simulink model "sistema_caotico"  (R2025b)
settings: Solver=ode4  StartTime=0.0  StopTime=5600  FixedStep=0.01  RelTol=1e-3
settings Model: Creator=Magallón  LastModifiedBy=aleja
settings SolverCC: AlgebraicLoopSolver=TrustRegion
settings OptimizationCC: ReuseModelBlockBuffer=off
settings DebuggingCC: UnconnectedInputMsg=warning  UnconnectedOutputMsg=warning  UnconnectedLineMsg=warning
settings ModelReferenceCC: EnableRefExpFcnMdlSchedulingChecks=on
settings SFSimCC: CustomCodeUndefinedFunction=UseInterfaceOnly
settings RTWCC: GPUComputeCapability=3.5

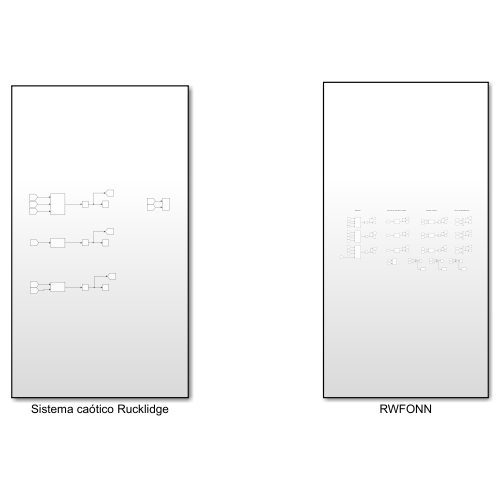
[thumbnail: Simulink's stored preview of the top-level diagram]
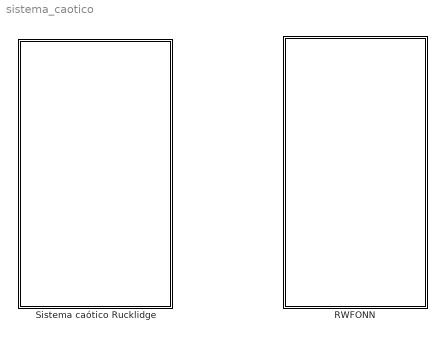
== system sistema_caotico ==
  RWFONN : Subsystem
  Sistema caótico Rucklidge : Subsystem

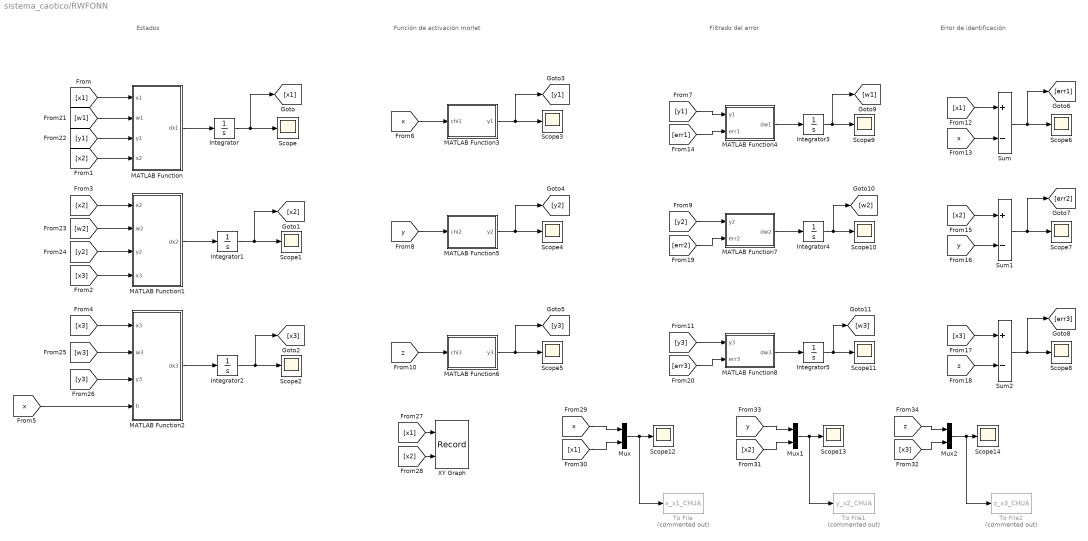
== system sistema_caotico/RWFONN ==
  note: Estados
  note: Función de activación morlet
  note: Filtrado del error
  note: Error de identificación
  Integrator : Integrator  InitialCondition=0.15
  Integrator1 : Integrator  InitialCondition=0.18
  Integrator2 : Integrator  InitialCondition=0.2
  Integrator3 : Integrator
  Integrator4 : Integrator
  Integrator5 : Integrator
  MATLAB Function : MATLAB Function  TreatAsAtomicUnit=on
  MATLAB Function1 : MATLAB Function  TreatAsAtomicUnit=on
  MATLAB Function2 : MATLAB Function  TreatAsAtomicUnit=on
  MATLAB Function3 : MATLAB Function  TreatAsAtomicUnit=on
  MATLAB Function4 : MATLAB Function  TreatAsAtomicUnit=on
  MATLAB Function5 : MATLAB Function  TreatAsAtomicUnit=on
  MATLAB Function6 : MATLAB Function  TreatAsAtomicUnit=on
  MATLAB Function7 : MATLAB Function  TreatAsAtomicUnit=on
  MATLAB Function8 : MATLAB Function  TreatAsAtomicUnit=on
  Mux : Mux  Inputs=2
  Mux1 : Mux  Inputs=2
  Mux2 : Mux  Inputs=2
  Scope{,1..14} (15 alike) : Scope
      Scope settings: ActiveDisplayYMinimum=-3.64404  ActiveDisplayYMaximum=3.74396  DataLoggingVariableName=ScopeData2
      Scope1 settings: ActiveDisplayYMinimum=-0.62184  ActiveDisplayYMaximum=0.61899  DataLoggingVariableName=ScopeData3
      Scope10 settings: DataLoggingVariableName=ScopeData8
      Scope11 settings: DataLoggingVariableName=ScopeData9
      Scope12 settings: ActiveDisplayYMinimum=-12.72999233304083  ActiveDisplayYMaximum=12.691522590822398  DataLoggingVariableName=ScopeData10
      Scope13 settings: ActiveDisplayYMinimum=-1.93605  ActiveDisplayYMaximum=1.07127  DataLoggingVariableName=ScopeData11
      Scope14 settings: ActiveDisplayYMinimum=-0.11038  ActiveDisplayYMaximum=0.33307  DataLoggingVariableName=ScopeData12
      Scope2 settings: ActiveDisplayYMinimum=-9.41356  ActiveDisplayYMaximum=31.13321  DataLoggingVariableName=ScopeData4
      Scope3 settings: ActiveDisplayYMinimum=0.95913  ActiveDisplayYMaximum=1.00454
      Scope4 settings: DataLoggingVariableName=ScopeData2
      Scope5 settings: DataLoggingVariableName=ScopeData3
      Scope6 settings: ActiveDisplayYMinimum=-0.066577278149702268  ActiveDisplayYMaximum=0.0653822169395355  DataLoggingVariableName=ScopeData4
      Scope7 settings: ActiveDisplayYMinimum=-0.00783  ActiveDisplayYMaximum=0.00738  DataLoggingVariableName=ScopeData5
      Scope8 settings: ActiveDisplayYMinimum=-1.2415250279876853  ActiveDisplayYMaximum=1.9808572797287463  DataLoggingVariableName=ScopeData6
      Scope9 settings: ActiveDisplayYMinimum=-1.38218  ActiveDisplayYMaximum=2.36611  DataLoggingVariableName=ScopeData7
  Sum : Sum  Inputs=+-
  Sum1 : Sum  Inputs=+-
  Sum2 : Sum  Inputs=+-
  To File : ToFile  Commented=on  Filename=x_x1_CHUA  MatrixName=x_x1_CHUA
  To File1 : ToFile  Commented=on  Filename=y_x2_CHUA  MatrixName=y_x2_CHUA
  To File2 : ToFile  Commented=on  Filename=z_x3_CHUA  MatrixName=z_x3_CHUA
  XY Graph : Record  NumPorts=2.0  FileSettingsInternal="{\"entries\":[{\"content\":{\"excelSettings\":{\"content\":{},\"type\":\"Streamout.ExcelSettings\"},\"parquetSettings\":{\"content\":{},\"type\":\"Streamout.ParquetSettings\"}},\"type\":\"Streamout.FileSettingStorage\",\"uuid\":\"\"}],\"packageUris\":[\"http:\\/\\/schema.mathworks.com\\/mf0\\/streamout_blocks\\/R2020a\"],\"version\":\"1.0\"}"  FrameSettings=[0, 0]  Layout=[1 1]  SignalsInternal="{\"entries\":[{\"content\":{\"signals\":[{\"content\":{\"blockPath\":[],\"dimensions\":[1],\"domain\":\"\",\"lineColor\":\"#a2142f\",\"plots\":[ 1 ],\"port\":1,\"signalID\":1,\"signalName\":\"From27\"},\"type\":\"RecordBlkView.Signal\",\"uuid\":\"\"},{\"content\":{\"blockPath\":[],\"dimensions\":[1],\"domain\":\"\",\"lineColor\":\"#139fff\",\"plots\":[ 1 ],\"port\":2,\"signalID\":2,\"signalName\":\"From28\"},\"type\":\"RecordBlkView.Signal\",\"uuid\":\"\"}]},\"type\":\"RecordBlkView.InputSignals\",\"uuid\":\"\"}],\"packageUris\":[\"http:\\/\\/schema.mathworks.com\\/mf0\\/streamout_blocks\\/R2020a\"],\"version\":\"1.0\"}"  VisualizationBindings="{\"xyplotplugin\":{\"info\":[{\"series\":[{\"bindingParametersList\":[{\"parameter\":\"X-Axis\",\"signalID\":1,\"signalName\":\"From27\"},{\"parameter\":\"Y-Axis\",\"signalID\":2,\"signalName\":\"From28\"}],\"seriesID\":0}],\"subplotID\":1}]}}"  CompatibilityTag=XY
  wires:
  MATLAB Function/1(dx1) -> Integrator/1
  MATLAB Function1/1(dx2) -> Integrator1/1
  MATLAB Function2/1(dx3) -> Integrator2/1
  Integrator/1 -> [x1], Scope/1
  Integrator1/1 -> [x2], Scope1/1
  Integrator2/1 -> [x3], Scope2/1
  [x1] -> MATLAB Function/1(x1)
  [x2] -> MATLAB Function/4(x2)
  [x3] -> MATLAB Function1/4(x3)
  [x2] -> MATLAB Function1/1(x2)
  [x3] -> MATLAB Function2/1(x3)
  MATLAB Function3/1(y1) -> [y1], Scope3/1
  [y1] -> MATLAB Function4/1(y1)
  MATLAB Function5/1(y2) -> Scope4/1, [y2]
  MATLAB Function6/1(y3) -> [y3], Scope5/1
  [y2] -> MATLAB Function7/1(y2)
  [y3] -> MATLAB Function8/1(y3)
  [x1] -> Sum/1
  Sum/1 -> [err1], Scope6/1
  [err1] -> MATLAB Function4/2(err1)
  Sum1/1 -> Scope7/1, [err2]
  [x2] -> Sum1/1
  [x3] -> Sum2/1
  Sum2/1 -> [err3], Scope8/1
  [err2] -> MATLAB Function7/2(err2)
  [err3] -> MATLAB Function8/2(err3)
  MATLAB Function4/1(dw1) -> Integrator3/1
  MATLAB Function7/1(dw2) -> Integrator4/1
  MATLAB Function8/1(dw3) -> Integrator5/1
  Integrator3/1 -> [w1], Scope9/1
  Integrator4/1 -> [w2], Scope10/1
  Integrator5/1 -> [w3], Scope11/1
  [w1] -> MATLAB Function/2(w1)
  [y1] -> MATLAB Function/3(y1)
  [w2] -> MATLAB Function1/2(w2)
  [y2] -> MATLAB Function1/3(y2)
  [w3] -> MATLAB Function2/2(w3)
  [y3] -> MATLAB Function2/3(y3)
  [x] -> Mux/1
  [x1] -> Mux/2
  Mux/1 -> To File/1, Scope12/1
  Mux1/1 -> To File1/1, Scope13/1
  [x2] -> Mux1/2
  [y] -> Mux1/1
  [z] -> Mux2/1
  [x3] -> Mux2/2
  Mux2/1 -> To File2/1, Scope14/1
  [x] -> Sum/2
  [y] -> Sum1/2
  [z] -> Sum2/2
  [x] -> MATLAB Function3/1(chi1)
  [y] -> MATLAB Function5/1(chi2)
  [z] -> MATLAB Function6/1(chi3)
  [x] -> MATLAB Function2/4(b)
  [x1] -> XY Graph/1
  [x2] -> XY Graph/2

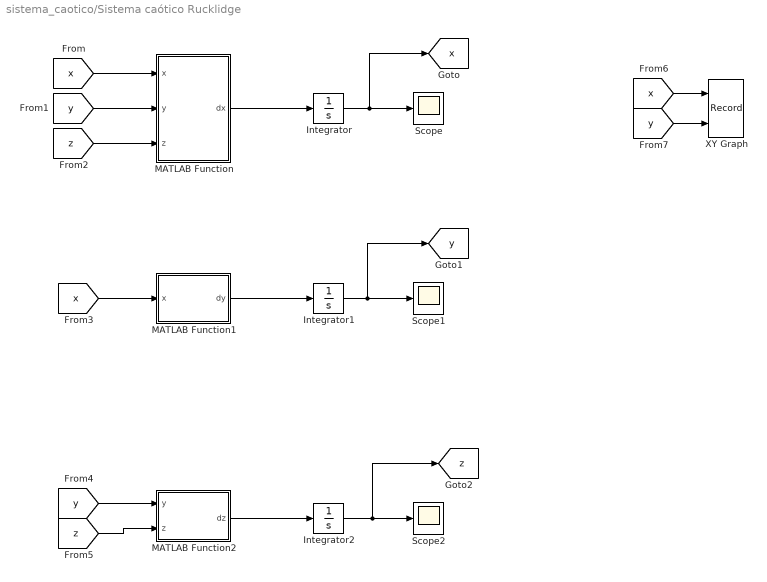
== system sistema_caotico/Sistema caótico Rucklidge ==
  Integrator : Integrator  InitialCondition=0.1
  Integrator1 : Integrator  InitialCondition=0.1
  Integrator2 : Integrator  InitialCondition=0.1
  MATLAB Function : MATLAB Function  TreatAsAtomicUnit=on
  MATLAB Function1 : MATLAB Function  TreatAsAtomicUnit=on
  MATLAB Function2 : MATLAB Function  TreatAsAtomicUnit=on
  Scope : Scope
      settings: ActiveDisplayYMinimum=-12.681396894045676  ActiveDisplayYMaximum=12.645318566895519
  Scope1 : Scope
      settings: ActiveDisplayYMinimum=-6.9478011204705394  ActiveDisplayYMaximum=6.95612990359057  DataLoggingVariableName=ScopeData2
  Scope2 : Scope
      settings: ActiveDisplayYMinimum=-1.845088493611583  ActiveDisplayYMaximum=17.286748359110742  DataLoggingVariableName=ScopeData3
  XY Graph : Record  NumPorts=2.0  FileSettingsInternal="{\"entries\":[{\"content\":{\"excelSettings\":{\"content\":{},\"type\":\"Streamout.ExcelSettings\"},\"parquetSettings\":{\"content\":{},\"type\":\"Streamout.ParquetSettings\"}},\"type\":\"Streamout.FileSettingStorage\",\"uuid\":\"\"}],\"packageUris\":[\"http:\\/\\/schema.mathworks.com\\/mf0\\/streamout_blocks\\/R2020a\"],\"version\":\"1.0\"}"  FrameSettings=[0, 0]  Layout=[1 1]  SignalsInternal="{\"entries\":[{\"content\":{\"signals\":[{\"content\":{\"blockPath\":[],\"dimensions\":[1],\"domain\":\"\",\"lineColor\":\"#edb120\",\"lineWidth\":2,\"plots\":[ 1 ],\"port\":1,\"signalID\":1,\"signalName\":\"From6\"},\"type\":\"RecordBlkView.Signal\",\"uuid\":\"\"},{\"content\":{\"blockPath\":[],\"dimensions\":[1],\"domain\":\"\",\"lineColor\":\"#7e2f8e\",\"lineWidth\":2,\"plots\":[ 1 ],\"port\":2,\"signalID\":2,\"signalName\":\"From7\"},\"type\":\"RecordBlkView.Signal\",\"uuid\":\"\"}]},\"type\":\"RecordBlkView.InputSignals\",\"uuid\":\"\"}],\"packageUris\":[\"http:\\/\\/schema.mathworks.com\\/mf0\\/streamout_blocks\\/R2020a\"],\"version\":\"1.0\"}"  VisualizationBindings="{\"xyplotplugin\":{\"info\":[{\"series\":[{\"bindingParametersList\":[{\"parameter\":\"X-Axis\",\"signalID\":1,\"signalName\":\"From6\"},{\"parameter\":\"Y-Axis\",\"signalID\":2,\"signalName\":\"From7\"}],\"seriesID\":0}],\"subplotID\":1}]}}"  CompatibilityTag=XY
  tag scope: x=global, y=global, z=global
  wires:
  MATLAB Function/1(dx) -> Integrator/1
  Integrator/1 -> [x], Scope/1
  MATLAB Function1/1(dy) -> Integrator1/1
  Integrator1/1 -> [y], Scope1/1
  MATLAB Function2/1(dz) -> Integrator2/1
  Integrator2/1 -> [z], Scope2/1
  [x] -> MATLAB Function/1(x)
  [y] -> MATLAB Function/2(y)
  [z] -> MATLAB Function/3(z)
  [x] -> MATLAB Function1/1(x)
  [y] -> MATLAB Function2/1(y)
  [z] -> MATLAB Function2/2(z)
  [x] -> XY Graph/1
  [y] -> XY Graph/2

== matlab function sistema_caotico/RWFONN/MATLAB Function ==
  data: x1 input; dx1 output; w1 input; y1 input; x2 input
function dx1 = fcn(x1,w1,y1,x2)
a1=5;
b1=5;

dx1 = -a1*x1+b1*w1*y1+x2;

== matlab function sistema_caotico/Sistema caótico Rucklidge/MATLAB Function2 ==
  data: y input; dz output; z input
function dz = fcn(y,z)

dz = y*y-z;

== matlab function sistema_caotico/RWFONN/MATLAB Function1 ==
  data: x2 input; w2 input; dx2 output; y2 input; x3 input
function dx2 = fcn(x2,w2,y2,x3)
a2=5;
b2=5;

dx2 = -a2*x2+b2*w2*y2+x3;

== matlab function sistema_caotico/RWFONN/MATLAB Function2 ==
  data: x3 input; dx3 output; w3 input; y3 input; b input
function dx3 = fcn(x3,w3,y3,b)
a3=5;
b3=5;

dx3 = -a3*x3+b3*w3*y3+b;

== matlab function sistema_caotico/RWFONN/MATLAB Function3 ==
  data: chi1 input; y1 output
function y1 = fcn(chi1)
lambda1=0.01;
beta1=100;

y1 = exp(-chi1^2/beta1)*cos(lambda1*chi1);
%function y1 = fcn(chi1)


%y1 = tanh(chi1);

== matlab function sistema_caotico/RWFONN/MATLAB Function4 ==
  data: y1 input; dw1 output; err1 input
function dw1 = fcn(y1,err1)
gamma1=5000;

dw1 = -gamma1*y1*err1;

== matlab function sistema_caotico/RWFONN/MATLAB Function5 ==
  data: chi2 input; y2 output
function y2 = fcn(chi2)
lambda2=0.01;
beta2=100;

y2 = exp(-chi2^2/beta2)*cos(lambda2*chi2);

== matlab function sistema_caotico/RWFONN/MATLAB Function6 ==
  data: chi3 input; y3 output
function y3 = fcn(chi3)
lambda3=0.01;
beta3=100;

y3 = exp(-chi3^2/beta3)*cos(lambda3*chi3);

== matlab function sistema_caotico/RWFONN/MATLAB Function7 ==
  data: y2 input; dw2 output; err2 input
function dw2 = fcn(y2,err2)
gamma2=5000;

dw2 = -gamma2*y2*err2;

== matlab function sistema_caotico/RWFONN/MATLAB Function8 ==
  data: y3 input; dw3 output; err3 input
function dw3 = fcn(y3,err3)
gamma3=5000;

dw3 = -gamma3*y3*err3;

== matlab function sistema_caotico/Sistema caótico Rucklidge/MATLAB Function ==
  data: x input; dx output; y input; z input
function dx = fcn(x,y,z)
a=2;           % VALOR DE ALFA 
b=6.7;

dx = -a*x+b*y-y*z;

== matlab function sistema_caotico/Sistema caótico Rucklidge/MATLAB Function1 ==
  data: x input; dy output
function dy = fcn(x)

dy = x;
